simulink model "Q9_W1"  (R2020b)
settings: Solver=VariableStepAuto  StartTime=0.0  StopTime=10.0  RelTol=1e-3
settings Model: Creator=hp  LastModifiedBy=hp

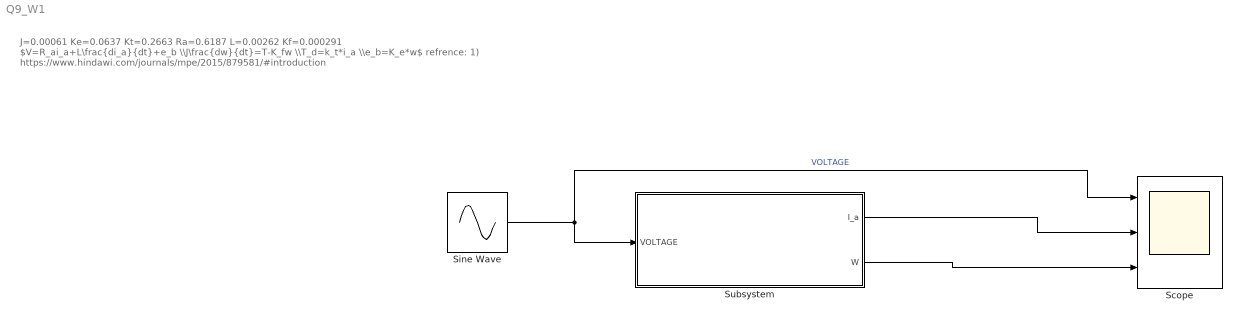
== system Q9_W1 ==
  note: J=0.00061
      | Ke=0.0637
      | Kt=0.2663
      | Ra=0.6187
      | L=0.00262
      | Kf=0.000291
      |
      | $V=R_ai_a+L\frac{di_a}{dt}+e_b \\J\frac{dw}{dt}=T-K_fw \\T_d=k_t*i_a \\e_b=K_e*w$
      | refrence:
      | 1) https://www.hindawi.com/journals/mpe/2015/879581/#introduction
  Scope : Scope  NumInputPorts=3
  Sine Wave : Sin  SampleTime=0
  Subsystem : Subsystem  TreatAsAtomicUnit=on
  wires:
  Sine Wave/1 -> Subsystem/1(VOLTAGE), Scope/1  "VOLTAGE"
  Subsystem/1(I_a) -> Scope/2
  Subsystem/2(W) -> Scope/3

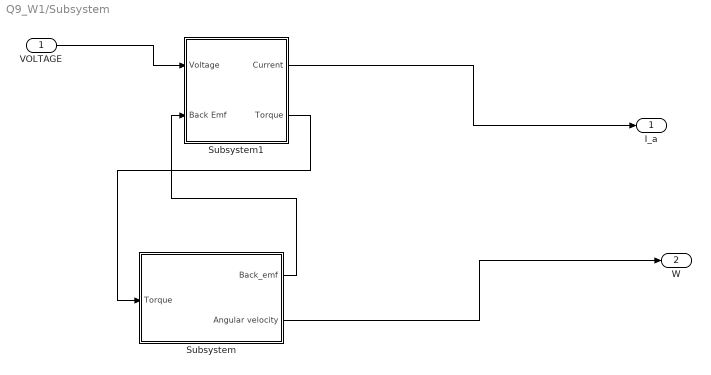
== system Q9_W1/Subsystem ==
  VOLTAGE : Inport
  Subsystem : Subsystem
  Subsystem1 : Subsystem
  I_a : Outport
  W : Outport  Port=2
  wires:
  Subsystem/2(Angular velocity) -> W/1
  VOLTAGE/1 -> Subsystem1/1(Voltage)
  Subsystem/1(Back_emf) -> Subsystem1/2(Back Emf)
  Subsystem1/1(Current) -> I_a/1
  Subsystem1/2(Torque) -> Subsystem/1(Torque)

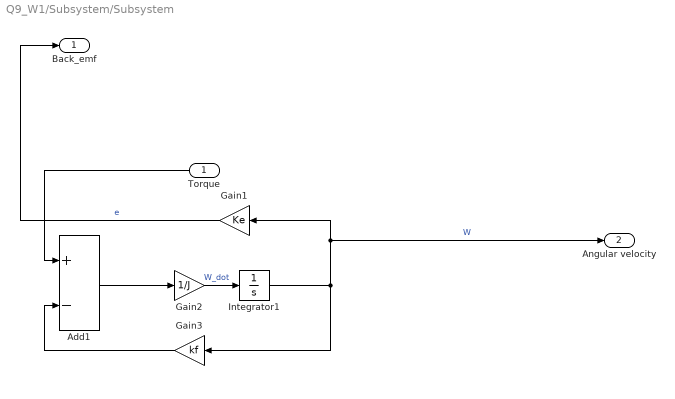
== system Q9_W1/Subsystem/Subsystem ==
  Torque : Inport
  Add1 : Sum  Inputs=+-
  Gain1 : Gain  Gain=Ke  mask{Ke=0.0637}
  Gain2 : Gain  Gain=1/J  mask{J=0.00061}
  Gain3 : Gain  Gain=kf  mask{kf=0.00291}
  Integrator1 : Integrator
  Back_emf : Outport
  Angular velocity : Outport  Port=2
  wires:
  Gain2/1 -> Integrator1/1  "W_dot"
  Add1/1 -> Gain2/1
  Integrator1/1 -> Angular velocity/1, Gain1/1, Gain3/1  "W"
  Gain3/1 -> Add1/2
  Gain1/1 -> Back_emf/1  "e"
  Torque/1 -> Add1/1

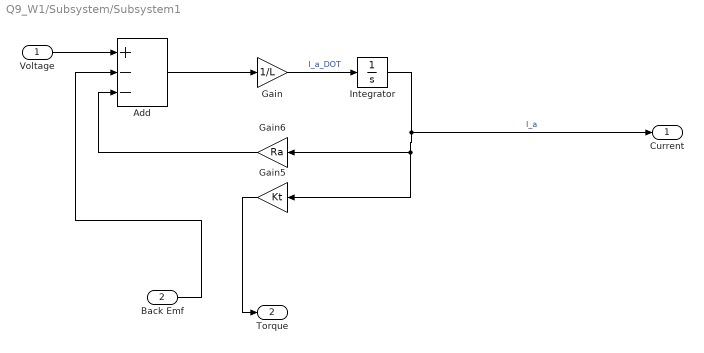
== system Q9_W1/Subsystem/Subsystem1 ==
  Voltage : Inport
  Back Emf : Inport  Port=2
  Add : Sum  Inputs=+--
  Gain : Gain  Gain=1/L  mask{L=0.00262}
  Gain5 : Gain  Gain=Kt  mask{Kt=0.2663}
  Gain6 : Gain  Gain=Ra  mask{Ra=0.6187}
  Integrator : Integrator
  Current : Outport
  Torque : Outport  Port=2
  wires:
  Voltage/1 -> Add/1
  Integrator/1 -> Current/1, Gain6/1, Gain5/1  "I_a"
  Gain/1 -> Integrator/1  "I_a_DOT"
  Gain6/1 -> Add/3
  Add/1 -> Gain/1
  Back Emf/1 -> Add/2
  Gain5/1 -> Torque/1
